simulink model "Ex2"  (Simulink 7.2)
settings: Solver=ode4  StartTime=0.0  StopTime=10  FixedStep=0.002  RelTol=1e-3
settings Model: Creator=controle  LastModifiedBy=controle  ExtModeTrigDuration=5000
settings SolverCC: PositivePriorityOrder=on
settings RTWCC: SystemTargetFile=quarc_windows.tlc  TemplateMakefile=quarc_default_tmf  Description=QUARC Win32 Target  ProcessScript=quarc_windows_make_rtw_hook
settings STFCustomTargetCC: TargetPreCompLibLocation=C:\DOCUME~1\ALLUSE~1\DADOSD~1\QUARC\lib\2008b\windows\release  SystemTargetFile=quarc_windows.tlc
settings GRTTargetCC: TargetPreCompLibLocation=C:\DOCUME~1\ALLUSE~1\DADOSD~1\QUARC\lib\2008b\windows\release  CompOptLevelCompliant=off  MatFileLogging=off  ExtMode=on  ExtModeMexFile=quarc_comm

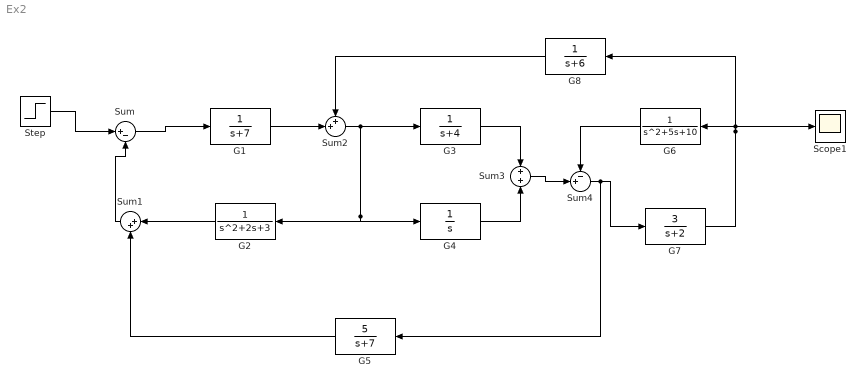
== system Ex2 ==
  G1 : TransferFcn  Denominator=[1 7]
  G2 : TransferFcn  Orientation=left  Denominator=[1 2 3]
  G3 : TransferFcn  Denominator=[1 4]
  G4 : TransferFcn  Denominator=[1 0]
  G5 : TransferFcn  Orientation=left  Numerator=[5]  Denominator=[1 7]
  G6 : TransferFcn  Orientation=left  Denominator=[1 5 10]
  G7 : TransferFcn  Numerator=[3]  Denominator=[1 2]
  G8 : TransferFcn  Orientation=left  Denominator=[1 6]
  Scope1 : Scope
      settings: YMin=0  YMax=700000
  Step : Step  SampleTime=0
  Sum : Sum  Inputs=|+-  OutDataType=sfix(16)  OutScaling=2^0
  Sum1 : Sum  Orientation=left  Inputs=|++  OutDataType=sfix(16)  OutScaling=2^0
  Sum2 : Sum  Inputs=++|  OutDataType=sfix(16)  OutScaling=2^0
  Sum3 : Sum  OutDataType=sfix(16)  OutScaling=2^0
  Sum4 : Sum  Inputs=-+|  OutDataType=sfix(16)  OutScaling=2^0
  wires:
  Sum/1 -> G1/1
  Sum1/1 -> Sum/2
  G2/1 -> Sum1/1
  G5/1 -> Sum1/2
  G1/1 -> Sum2/2
  G8/1 -> Sum2/1
  Sum2/1 -> G3/1, G2/1, G4/1
  G3/1 -> Sum3/1
  G4/1 -> Sum3/2
  Sum3/1 -> Sum4/2
  G6/1 -> Sum4/1
  Sum4/1 -> G7/1, G5/1
  G7/1 -> G8/1, G6/1, Scope1/1
  Step/1 -> Sum/1
